simulink model "quad_control_elev8_sAttit_training"  (Simulink 8.7)
settings: Solver=FixedStepAuto  StartTime=0.0  StopTime=20  FixedStep=0.01  RelTol=1e-3
InitFcn:
  | % --- Inner loop gains --------
  | %Kp_pitch = 2.5;   Kp_roll = 2.5;    Kp_yaw = 0.4;
  | %Ki_pitch = 0.06;  Ki_roll = 0.055; Ki_yaw = 0.095;
  | %Kd_pitch = 1.25; Kd_roll = 1.25;  Kd_yaw = 1.2;
  | % --------------------------
  | 
  | % --- Outer loop gains --------
  | P_X=9.44;   I_X=0.23; D_X=2.36;
  | P_Y=9.33;   I_Y=0.18; D_Y=1.54;
  | %P_Z = 32; I_Z = 5;  D_Z = 10;
  | % --------------------------
  | 
  | % --- Saturation limits --------
  | attit_upper_limit = 10;
  | attit_lower_limit = -10;
  | 
  | pos_upper_limit = 1;
  | pos_lower_limit = -1;
  | 
  | mvel_upper_limit = 30;
  | mvel_lower_limit = 5;
  | % --------------------------
  | 
  | %gera o valor do angulo
  | %aleatoreamente para o treinamendo
  | %de posicao
  | %rand_ang = pi + (-pi-pi).*rand(1,1);
  | %rand_altur = 1 + (3-1).*rand(1,1);
  | 
  | global clientID;
  | clientID=-1;
values from neighbouring files (symbols this model uses):
  D_Z = 35.7414524229    [workspace.mat]    (also in workspace_inner.mat = 20.4994; workspace_outer.mat = 19.0535228097)
  enable_gripper = 0    [CARLA_INNER_CONTROLLERS.m]    (also in CARLA_OUTER_CONTROLLERS.m; workspace_inner.mat; workspace_outer.mat)
  I_Z = 14.6020346537    [workspace.mat]    (also in workspace_inner.mat = 22.8237; workspace_outer.mat = 43.091018381)
  P_Z = 59.4468680841    [workspace.mat]    (also in workspace_inner.mat = 26.3889; workspace_outer.mat = 57.1774186981)
  rand_ang = pi + (-pi-pi).*rand    [CARLA_OUTER_CONTROLLERS.m]    (also in workspace.mat = 2.59590225137; workspace_outer.mat = -1.93159407417)
undefined symbols (not defined in the file or in its folder): Angular, Linear, sigbuilder_block
libraries: simulink_extras x4, dspsigops x4, robotlib x3, aerolibtransform2 x1
settings Model: Creator=kleber  LastModifiedBy=kleber
settings DataIOCC: LimitDataPoints=off
settings DebuggingCC: UnderspecifiedInitializationDetection=Simplified  MergeDetectMultiDrivingBlocksExec=error  SolverPrmCheckMsg=warning
settings ConfigComp: CovSFcnEnable=off

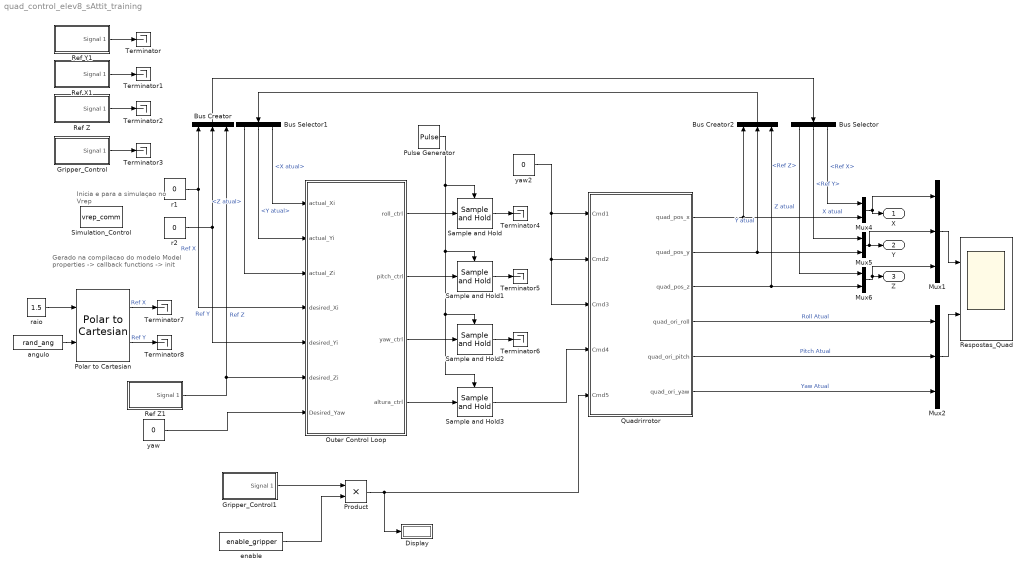
== system quad_control_elev8_sAttit_training ==
  note: Inicia e para a simulaçao no Vrep
  note: Gerado na compilacao do modelo
      | Model properties -> callback functions
      | -> init
  Bus Creator : BusCreator  Inputs=3
  Bus Creator2 : BusCreator  Inputs=3
  Bus Selector : BusSelector  OutputSignals=Ref Z,Ref Y,Ref X
  Bus Selector1 : BusSelector  OutputSignals=Z atual,Y atual,X atual
  Display : Display
  Gripper_Control : Subsystem  Tag=STV Subsys  LoadFcn=sigbuilder_block('load');  StartFcn=sigbuilder_block('start');  StopFcn=sigbuilder_block('stop');  ClipboardFcn=sigbuilder_block('clipboard');  mask(Sigbuilder block){}
      mask help: Sigbuilder GUI
      mask init:
      | if ~strcmp(get_param(bdroot(gcbh),'SimulationStatus'),'stopped') tuvar = sigbuilder_block('maskInit'); end
      settings: CopyFcn=sigbuilder_block('copy');  DeleteFcn=sigbuilder_block('delete');  ModelCloseFcn=sigbuilder_block('modelClose');  PreSaveFcn=sigbuilder_block('preSave');  PauseFcn=sigbuilder_block('pause')  ContinueFcn=sigbuilder_block('continue')  NameChangeFcn=sigbuilder_block('namechange');  OpenFcn=sigbuilder_block('open',[47.25 204 963.75 268.5 ]);  CloseFcn=sigbuilder_block('close');
      mask Display: plot(0,0,100,100,[10,10,40,40,10],[80,20,20,80,80],[40,10],[50,50], [40,27,10],[65,72,56],[40,25,25,10],[28,28,43,43]);
  Gripper_Control1 : Subsystem  Tag=STV Subsys  LoadFcn=sigbuilder_block('load');  StartFcn=sigbuilder_block('start');  StopFcn=sigbuilder_block('stop');  ClipboardFcn=sigbuilder_block('clipboard');  mask(Sigbuilder block){}
      mask help: Sigbuilder GUI
      mask init:
      | if ~strcmp(get_param(bdroot(gcbh),'SimulationStatus'),'stopped') tuvar = sigbuilder_block('maskInit'); end
      settings: CopyFcn=sigbuilder_block('copy');  DeleteFcn=sigbuilder_block('delete');  ModelCloseFcn=sigbuilder_block('modelClose');  PreSaveFcn=sigbuilder_block('preSave');  PauseFcn=sigbuilder_block('pause')  ContinueFcn=sigbuilder_block('continue')  NameChangeFcn=sigbuilder_block('namechange');  OpenFcn=sigbuilder_block('open',[47.25 138 956.25 246 ]);  CloseFcn=sigbuilder_block('close');
      mask Display: plot(0,0,100,100,[10,10,40,40,10],[80,20,20,80,80],[40,10],[50,50], [40,27,10],[65,72,56],[40,25,25,10],[28,28,43,43]);
  Mux1 : Mux  Inputs=3
  Mux2 : Mux  Inputs=3
  Mux4 : Mux  Inputs=2
  Mux5 : Mux  Inputs=2
  Mux6 : Mux  Inputs=2
  Outer Control Loop : Subsystem
  Polar to Cartesian : simulink_extras/Transformations/Polar to Cartesian
  Product : Product
  Pulse Generator : DiscretePulseGenerator  PulseType=Time based  Period=0.1  PulseWidth=10
  Quadrirrotor : Subsystem
  Ref X1 : Subsystem  Tag=STV Subsys  LoadFcn=sigbuilder_block('load');  StartFcn=sigbuilder_block('start');  StopFcn=sigbuilder_block('stop');  ClipboardFcn=sigbuilder_block('clipboard');  mask(Sigbuilder block){}
      mask help: Sigbuilder GUI
      mask init:
      | if ~strcmp(get_param(bdroot(gcbh),'SimulationStatus'),'stopped') tuvar = sigbuilder_block('maskInit'); end
      settings: CopyFcn=sigbuilder_block('copy');  DeleteFcn=sigbuilder_block('delete');  ModelCloseFcn=sigbuilder_block('modelClose');  PreSaveFcn=sigbuilder_block('preSave');  PauseFcn=sigbuilder_block('pause')  ContinueFcn=sigbuilder_block('continue')  NameChangeFcn=sigbuilder_block('namechange');  OpenFcn=sigbuilder_block('open',[62.25 205.5 902.25 227.25 ]);  CloseFcn=sigbuilder_block('close');
      mask Display: plot(0,0,100,100,[10,10,40,40,10],[80,20,20,80,80],[40,10],[50,50], [40,27,10],[65,72,56],[40,25,25,10],[28,28,43,43]);
  Ref Y1 : Subsystem  Tag=STV Subsys  LoadFcn=sigbuilder_block('load');  StartFcn=sigbuilder_block('start');  StopFcn=sigbuilder_block('stop');  ClipboardFcn=sigbuilder_block('clipboard');  mask(Sigbuilder block){}
      mask help: Sigbuilder GUI
      mask init:
      | if ~strcmp(get_param(bdroot(gcbh),'SimulationStatus'),'stopped') tuvar = sigbuilder_block('maskInit'); end
      settings: CopyFcn=sigbuilder_block('copy');  DeleteFcn=sigbuilder_block('delete');  ModelCloseFcn=sigbuilder_block('modelClose');  PreSaveFcn=sigbuilder_block('preSave');  PauseFcn=sigbuilder_block('pause')  ContinueFcn=sigbuilder_block('continue')  NameChangeFcn=sigbuilder_block('namechange');  OpenFcn=sigbuilder_block('open',[57.75 194.25 908.25 252 ]);  CloseFcn=sigbuilder_block('close');
      mask Display: plot(0,0,100,100,[10,10,40,40,10],[80,20,20,80,80],[40,10],[50,50], [40,27,10],[65,72,56],[40,25,25,10],[28,28,43,43]);
  Ref Z : Subsystem  Tag=STV Subsys  LoadFcn=sigbuilder_block('load');  StartFcn=sigbuilder_block('start');  StopFcn=sigbuilder_block('stop');  ClipboardFcn=sigbuilder_block('clipboard');  mask(Sigbuilder block){}
      mask help: Sigbuilder GUI
      mask init:
      | if ~strcmp(get_param(bdroot(gcbh),'SimulationStatus'),'stopped') tuvar = sigbuilder_block('maskInit'); end
      settings: CopyFcn=sigbuilder_block('copy');  DeleteFcn=sigbuilder_block('delete');  ModelCloseFcn=sigbuilder_block('modelClose');  PreSaveFcn=sigbuilder_block('preSave');  PauseFcn=sigbuilder_block('pause')  ContinueFcn=sigbuilder_block('continue')  NameChangeFcn=sigbuilder_block('namechange');  OpenFcn=sigbuilder_block('open',[41.25 0 973.5 255 ]);  CloseFcn=sigbuilder_block('close');
      mask Display: plot(0,0,100,100,[10,10,40,40,10],[80,20,20,80,80],[40,10],[50,50], [40,27,10],[65,72,56],[40,25,25,10],[28,28,43,43]);
  Ref Z1 : Subsystem  Tag=STV Subsys  LoadFcn=sigbuilder_block('load');  StartFcn=sigbuilder_block('start');  StopFcn=sigbuilder_block('stop');  ClipboardFcn=sigbuilder_block('clipboard');  mask(Sigbuilder block){}
      mask help: Sigbuilder GUI
      mask init:
      | if ~strcmp(get_param(bdroot(gcbh),'SimulationStatus'),'stopped') tuvar = sigbuilder_block('maskInit'); end
      settings: CopyFcn=sigbuilder_block('copy');  DeleteFcn=sigbuilder_block('delete');  ModelCloseFcn=sigbuilder_block('modelClose');  PreSaveFcn=sigbuilder_block('preSave');  PauseFcn=sigbuilder_block('pause')  ContinueFcn=sigbuilder_block('continue')  NameChangeFcn=sigbuilder_block('namechange');  OpenFcn=sigbuilder_block('open',[45 0 979.5 343.5 ]);  CloseFcn=sigbuilder_block('close');
      mask Display: plot(0,0,100,100,[10,10,40,40,10],[80,20,20,80,80],[40,10],[50,50], [40,27,10],[65,72,56],[40,25,25,10],[28,28,43,43]);
  Respostas_Quad : Scope  NumInputPorts=2
  Sample and Hold{,1..3} (4 alike) : dspsigops/Sample and Hold  trig=Rising edge  initCond=0  latchinput=off
  Simulation_Control : S-Function  FunctionName=vrep_comm  SFunctionDeploymentMode=off  EnableBusSupport=off
  Terminator{,1..8} (9 alike) : Terminator
  angulo : Constant  Value=rand_ang
  enable : Constant  Value=enable_gripper
  r1 : Constant  Value=0
  r2 : Constant  Value=0
  raio : Constant  Value=1.5
  yaw : Constant  Value=0
  yaw2 : Constant  Value=0
  X : Outport
  Y : Outport  Port=2
  Z : Outport  Port=3
  wires:
  Mux1/1 -> Respostas_Quad/1
  Mux2/1 -> Respostas_Quad/2
  Quadrirrotor/5(quad_ori_pitch) -> Mux2/2  "Pitch Atual"
  Quadrirrotor/4(quad_ori_roll) -> Mux2/1  "Roll Atual"
  Quadrirrotor/1(quad_pos_x) -> Bus Creator2/1, Mux4/2  "X atual"
  Quadrirrotor/3(quad_pos_z) -> Bus Creator2/3, Mux6/2  "Z atual"
  Quadrirrotor/6(quad_ori_yaw) -> Mux2/3  "Yaw Atual"
  yaw2/1 -> Quadrirrotor/1(Cmd1), Quadrirrotor/2(Cmd2), Quadrirrotor/3(Cmd3)
  yaw/1 -> Outer Control Loop/7(Desired_Yaw)
  Pulse Generator/1 -> Sample and Hold/Trigger, Sample and Hold2/Trigger, Sample and Hold3/Trigger, Sample and Hold1/Trigger
  Outer Control Loop/4(altura_ctrl) -> Sample and Hold3/1
  Mux4/1 -> X/1, Mux1/1
  Mux5/1 -> Y/1, Mux1/2
  Mux6/1 -> Mux1/3, Z/1
  Outer Control Loop/3(yaw_ctrl) -> Sample and Hold2/1
  Outer Control Loop/2(pitch_ctrl) -> Sample and Hold1/1
  Outer Control Loop/1(roll_ctrl) -> Sample and Hold/1
  r2/1 -> Outer Control Loop/5(desired_Yi), Bus Creator/2  "Ref Y"
  r1/1 -> Outer Control Loop/4(desired_Xi), Bus Creator/1  "Ref X"
  Quadrirrotor/2(quad_pos_y) -> Bus Creator2/2, Mux5/2  "Y atual"
  Sample and Hold3/1 -> Quadrirrotor/4(Cmd4)
  angulo/1 -> Polar to Cartesian/2
  raio/1 -> Polar to Cartesian/1
  Gripper_Control1/1(Signal 1) -> Product/1
  enable/1 -> Product/2
  Ref Y1/1(Signal 1) -> Terminator/1
  Ref X1/1(Signal 1) -> Terminator1/1
  Ref Z/1(Signal 1) -> Terminator2/1
  Gripper_Control/1(Signal 1) -> Terminator3/1
  Ref Z1/1(Signal 1) -> Outer Control Loop/6(desired_Zi), Bus Creator/3  "Ref Z"
  Bus Creator/1 -> Bus Selector/1
  Bus Selector/3 -> Mux4/1  "<Ref X>"
  Bus Selector/2 -> Mux5/1  "<Ref Y>"
  Bus Selector/1 -> Mux6/1  "<Ref Z>"
  Bus Selector1/3 -> Outer Control Loop/1(actual_Xi)  "<X atual>"
  Bus Selector1/2 -> Outer Control Loop/2(actual_Yi)  "<Y atual>"
  Bus Selector1/1 -> Outer Control Loop/3(actual_Zi)  "<Z atual>"
  Bus Creator2/1 -> Bus Selector1/1
  Product/1 -> Display/1, Quadrirrotor/5(Cmd5)
  Sample and Hold/1 -> Terminator4/1
  Sample and Hold1/1 -> Terminator5/1
  Sample and Hold2/1 -> Terminator6/1
  Polar to Cartesian/1 -> Terminator7/1  "Ref X"
  Polar to Cartesian/2 -> Terminator8/1  "Ref Y"

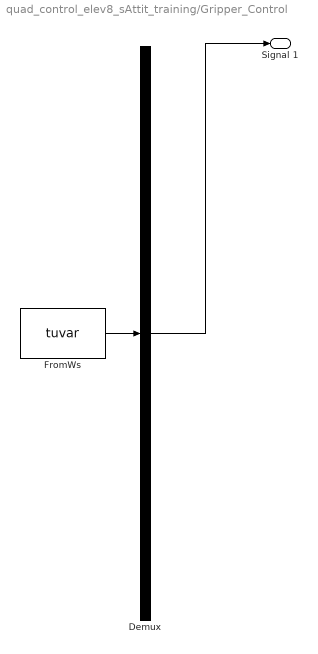
== system quad_control_elev8_sAttit_training/Gripper_Control ==
  Demux : Demux  Tag=STV Demux  Outputs=1
  FromWs : FromWorkspace  Tag=STV FromWs  VariableName=tuvar  SampleTime=0  SigBuilderData=DataTag0  VnvData=DataTag1
      SigBuilderData=|
      | common.afterFinalStr = 'Extrapolate'
      | common.sampleTime = 0
      | dataSet.timeRange = [0 250]
      | dataSet.name = 'Group 1'
      | sbobj.Name = 'Signal Builder'
      | sbobj.Groups.Name = 'Group 1'
      | sbobj.Groups.Signals.Name = 'Signal 1'
      | sbobj.Groups.Signals.XData = [0 35 35 100 100 155 155 220 220 250]
      | sbobj.Groups.Signals.YData = [0 0 1 1 0 0 1 1 0 0]
      | sbobj.Groups.TimeRange = [0 250]
  Signal 1 : Outport  Tag=STV Outport
  wires:
  FromWs/1 -> Demux/1
  Demux/1 -> Signal 1/1

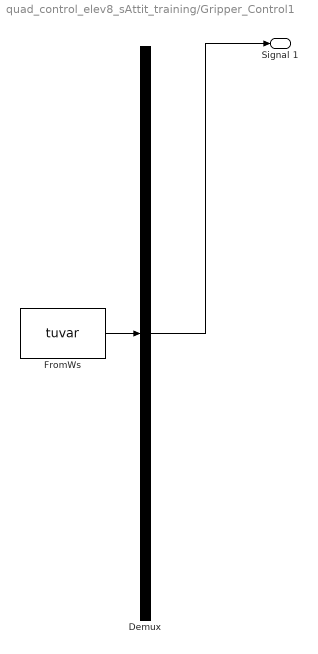
== system quad_control_elev8_sAttit_training/Gripper_Control1 ==
  Demux : Demux  Tag=STV Demux  Outputs=1
  FromWs : FromWorkspace  Tag=STV FromWs  VariableName=tuvar  SampleTime=0  SigBuilderData=DataTag2  VnvData=DataTag3
      SigBuilderData=|
      | common.afterFinalStr = 'Extrapolate'
      | common.sampleTime = 0
      | dataSet.timeRange = [0 40]
      | dataSet.name = 'Group 1'
      | sbobj.Name = 'Signal Builder'
      | sbobj.Groups.Name = 'Group 1'
      | sbobj.Groups.Signals.Name = 'Signal 1'
      | sbobj.Groups.Signals.XData = [0 22.5 22.5 40]
      | sbobj.Groups.Signals.YData = [1 1 0 0]
      | sbobj.Groups.TimeRange = [0 40]
  Signal 1 : Outport  Tag=STV Outport
  wires:
  Demux/1 -> Signal 1/1
  FromWs/1 -> Demux/1

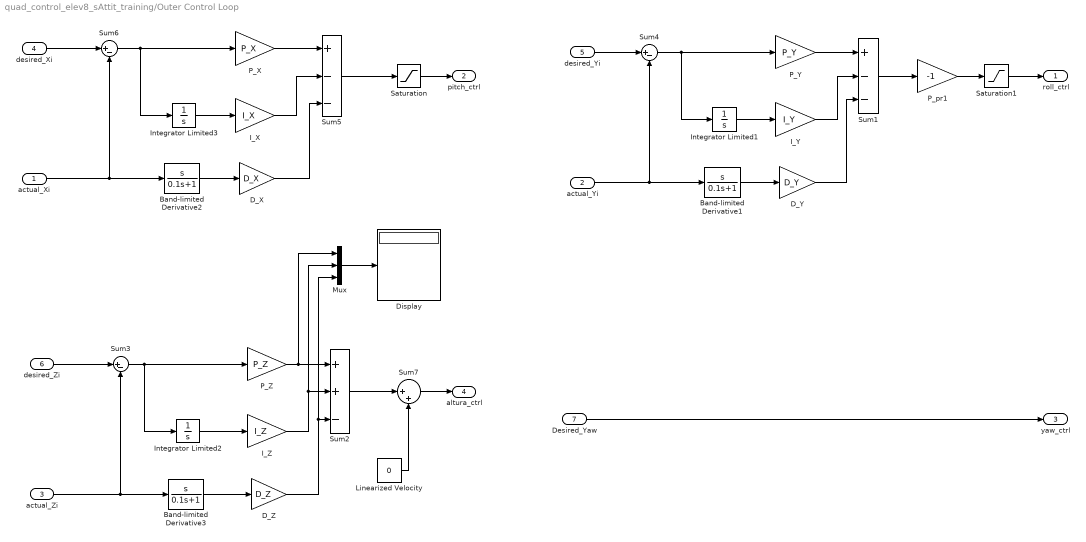
== system quad_control_elev8_sAttit_training/Outer Control Loop ==
  actual_Xi : Inport
  actual_Yi : Inport  Port=2
  actual_Zi : Inport  Port=3
  desired_Xi : Inport  Port=4
  desired_Yi : Inport  Port=5
  desired_Zi : Inport  Port=6
  Desired_Yaw : Inport  Port=7
  Band-limited Derivative1 : TransferFcn  Numerator=[1 0]  Denominator=[0.1 1]
  Band-limited Derivative2 : TransferFcn  Numerator=[1 0]  Denominator=[0.1 1]
  Band-limited Derivative3 : TransferFcn  Numerator=[1 0]  Denominator=[0.1 1]
  D_X : Gain  Gain=D_X
  D_Y : Gain  Gain=D_Y
  D_Z : Gain  Gain=D_Z
  Display : Display
  I_X : Gain  Gain=I_X
  I_Y : Gain  Gain=I_Y
  I_Z : Gain  Gain=I_Z
  Integrator Limited1 : Integrator  LimitOutput=on  UpperSaturationLimit=0.5  LowerSaturationLimit=-0.5
  Integrator Limited2 : Integrator  LimitOutput=on  UpperSaturationLimit=10  LowerSaturationLimit=0
  Integrator Limited3 : Integrator  LimitOutput=on  UpperSaturationLimit=0.5  LowerSaturationLimit=-0.5
  Linearized Velocity : Constant  Value=0
  Mux : Mux  Inputs=3
  P_X : Gain  Gain=P_X
  P_Y : Gain  Gain=P_Y
  P_Z : Gain  Gain=P_Z
  P_pr1 : Gain  Gain=-1
  Saturation : Saturate  UpperLimit=2  LowerLimit=-2
  Saturation1 : Saturate  UpperLimit=2  LowerLimit=-2
  Sum1 : Sum  Inputs=+--
  Sum2 : Sum  Inputs=++-
  Sum3 : Sum  Inputs=|+-
  Sum4 : Sum  Inputs=|+-
  Sum5 : Sum  Inputs=+--
  Sum6 : Sum  Inputs=|+-
  Sum7 : Sum  Inputs=|++
  roll_ctrl : Outport
  pitch_ctrl : Outport  Port=2
  yaw_ctrl : Outport  Port=3
  altura_ctrl : Outport  Port=4
  wires:
  Sum7/1 -> altura_ctrl/1
  Desired_Yaw/1 -> yaw_ctrl/1
  Sum1/1 -> P_pr1/1
  Sum2/1 -> Sum7/1
  Linearized Velocity/1 -> Sum7/2
  Sum5/1 -> Saturation/1
  Saturation/1 -> pitch_ctrl/1
  P_pr1/1 -> Saturation1/1
  Saturation1/1 -> roll_ctrl/1
  Mux/1 -> Display/1
  Sum3/1 -> Integrator Limited2/1, P_Z/1
  P_Z/1 -> Mux/1, Sum2/1
  D_Z/1 -> Mux/3, Sum2/3
  Band-limited Derivative3/1 -> D_Z/1
  I_Z/1 -> Mux/2, Sum2/2
  Sum6/1 -> Integrator Limited3/1, P_X/1
  Integrator Limited3/1 -> I_X/1
  P_X/1 -> Sum5/1
  D_X/1 -> Sum5/3
  actual_Xi/1 -> Band-limited Derivative2/1, Sum6/2
  Band-limited Derivative2/1 -> D_X/1
  desired_Xi/1 -> Sum6/1
  I_X/1 -> Sum5/2
  Integrator Limited2/1 -> I_Z/1
  Sum4/1 -> Integrator Limited1/1, P_Y/1
  Integrator Limited1/1 -> I_Y/1
  P_Y/1 -> Sum1/1
  D_Y/1 -> Sum1/3
  actual_Yi/1 -> Sum4/2, Band-limited Derivative1/1
  Band-limited Derivative1/1 -> D_Y/1
  desired_Yi/1 -> Sum4/1
  I_Y/1 -> Sum1/2
  actual_Zi/1 -> Sum3/2, Band-limited Derivative3/1
  desired_Zi/1 -> Sum3/1

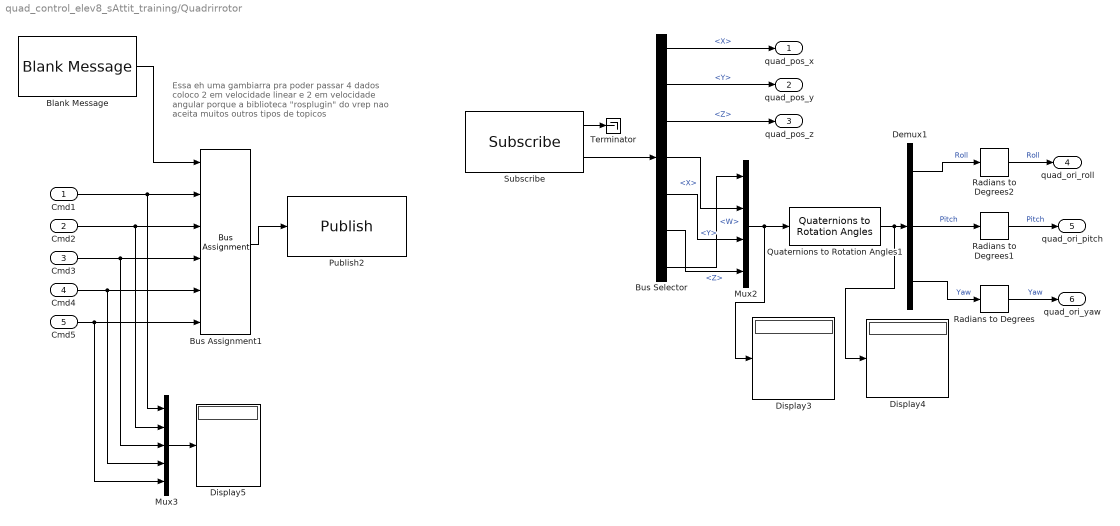
== system quad_control_elev8_sAttit_training/Quadrirrotor ==
  note: Essa eh uma gambiarra pra poder passar 4 dados coloco 2 em velocidade linear e 2 em velocidade angular porque a biblioteca "rosplugin" do vrep nao aceita muitos outros tipos de topicos
  Cmd1 : Inport
  Cmd2 : Inport  Port=2
  Cmd3 : Inport  Port=3
  Cmd4 : Inport  Port=4
  Cmd5 : Inport  Port=5
  Blank Message : robotlib/Blank Message  SourceLibraryInfo=This block requires Robotics System Toolbox  messageType=geometry_msgs/Twist  SampleTime=inf
  Bus Assignment1 : BusAssignment  DialogController=Simulink.DDGSource_BusAssignment  AssignedSignals=Linear.X,Linear.Y,Angular.X,Angular.Y,Angular.Z
  Bus Selector : BusSelector  OutputSignals=Pose.Position.X,Pose.Position.Y,Pose.Position.Z,Pose.Orientation.X,Pose.Orientation.Y,Pose.Orientation.Z,Pose.Orientation.W
  Demux1 : Demux  Outputs=3
  Display3 : Display
  Display4 : Display
  Display5 : Display
  Mux2 : Mux
  Mux3 : Mux  Inputs=5
  Publish2 : robotlib/Publish  SourceLibraryInfo=This block requires Robotics System Toolbox  topicSource=Select from ROS network  topic=/control_signals  messageType=geometry_msgs/Twist  messageQueueLength=105
  Quaternions to Rotation Angles1 : aerolibtransform2/Quaternions to Rotation Angles  rotationOrder=XYZ
  Radians to Degrees : simulink_extras/Transformations/Radians to Degrees
  Radians to Degrees1 : simulink_extras/Transformations/Radians to Degrees
  Radians to Degrees2 : simulink_extras/Transformations/Radians to Degrees
  Subscribe : robotlib/Subscribe  SourceLibraryInfo=This block requires Robotics System Toolbox  topicSource=Select from ROS network  topic=/quad_pos_ang  messageType=geometry_msgs/PoseStamped  sampleTime=-1  messageQueueLength=51
  Terminator : Terminator
  quad_pos_x : Outport
  quad_pos_y : Outport  Port=2
  quad_pos_z : Outport  Port=3
  quad_ori_roll : Outport  Port=4
  quad_ori_pitch : Outport  Port=5
  quad_ori_yaw : Outport  Port=6
  wires:
  Cmd1/1 -> Mux3/1, Bus Assignment1/2
  Bus Selector/1 -> quad_pos_x/1  "<X>"
  Bus Selector/2 -> quad_pos_y/1  "<Y>"
  Bus Selector/3 -> quad_pos_z/1  "<Z>"
  Radians to Degrees2/1 -> quad_ori_roll/1  "Roll"
  Radians to Degrees1/1 -> quad_ori_pitch/1  "Pitch"
  Radians to Degrees/1 -> quad_ori_yaw/1  "Yaw"
  Demux1/3 -> Radians to Degrees/1  "Yaw"
  Demux1/2 -> Radians to Degrees1/1  "Pitch"
  Demux1/1 -> Radians to Degrees2/1  "Roll"
  Bus Assignment1/1 -> Publish2/1
  Blank Message/1 -> Bus Assignment1/1
  Subscribe/2 -> Bus Selector/1
  Subscribe/1 -> Terminator/1
  Bus Selector/5 -> Mux2/3  "<Y>"
  Bus Selector/6 -> Mux2/4  "<Z>"
  Bus Selector/7 -> Mux2/1  "<W>"
  Mux2/1 -> Quaternions to Rotation Angles1/1, Display3/1
  Bus Selector/4 -> Mux2/2  "<X>"
  Cmd3/1 -> Mux3/3, Bus Assignment1/4
  Cmd4/1 -> Bus Assignment1/5, Mux3/4
  Quaternions to Rotation Angles1/1 -> Display4/1, Demux1/1
  Mux3/1 -> Display5/1
  Cmd2/1 -> Mux3/2, Bus Assignment1/3
  Cmd5/1 -> Bus Assignment1/6, Mux3/5

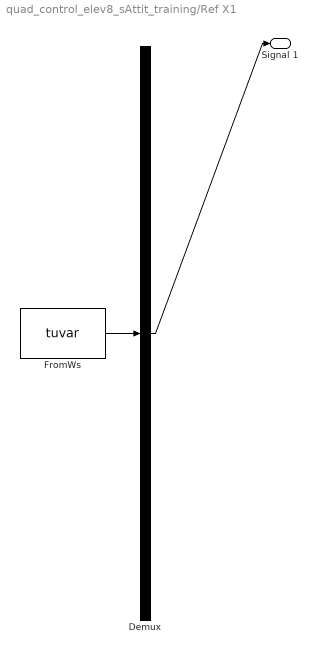
== system quad_control_elev8_sAttit_training/Ref X1 ==
  Demux : Demux  Tag=STV Demux  Outputs=1
  FromWs : FromWorkspace  Tag=STV FromWs  VariableName=tuvar  SampleTime=0  SigBuilderData=DataTag4  VnvData=DataTag5
      SigBuilderData=|
      | common.afterFinalStr = 'Extrapolate'
      | common.sampleTime = 0
      | dataSet.timeRange = [0 250]
      | dataSet.name = 'Group 1'
      | sbobj.Name = 'Signal Builder'
      | sbobj.Groups.Name = 'Group 1'
      | sbobj.Groups.Signals.Name = 'Signal 1'
      | sbobj.Groups.Signals.XData = [0 10 110 130 250]
      | sbobj.Groups.Signals.YData = [0 1 1 1.5 1.5]
      | sbobj.Groups.TimeRange = [0 250]
  Signal 1 : Outport  Tag=STV Outport
  wires:
  FromWs/1 -> Demux/1
  Demux/1 -> Signal 1/1

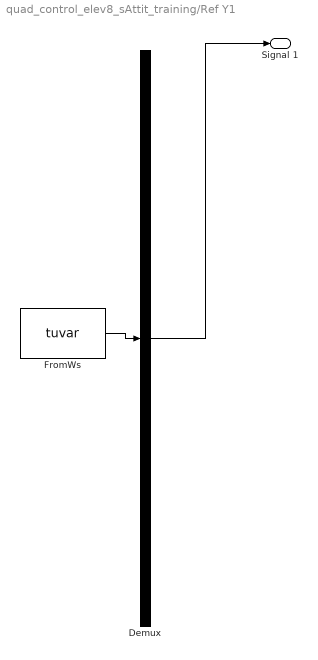
== system quad_control_elev8_sAttit_training/Ref Y1 ==
  Demux : Demux  Tag=STV Demux  Outputs=1
  FromWs : FromWorkspace  Tag=STV FromWs  VariableName=tuvar  SampleTime=0  SigBuilderData=DataTag6  VnvData=DataTag7
      SigBuilderData=|
      | common.afterFinalStr = 'Extrapolate'
      | common.sampleTime = 0
      | dataSet.timeRange = [0 250]
      | dataSet.name = 'Group 1'
      | sbobj.Name = 'Signal Builder'
      | sbobj.Groups.Name = 'Group 1'
      | sbobj.Groups.Signals.Name = 'Signal 1'
      | sbobj.Groups.Signals.XData = [0 10 50 70 105 130 170 190 250]
      | sbobj.Groups.Signals.YData = [0 0.5 0.5 2.5 2.5 0.5 0.5 2.5 2.5]
      | sbobj.Groups.TimeRange = [0 250]
  Signal 1 : Outport  Tag=STV Outport
  wires:
  Demux/1 -> Signal 1/1
  FromWs/1 -> Demux/1

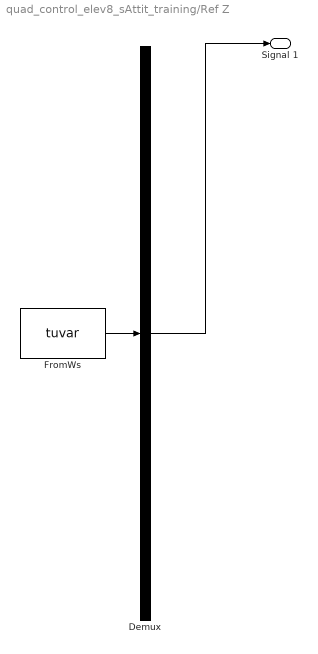
== system quad_control_elev8_sAttit_training/Ref Z ==
  Demux : Demux  Tag=STV Demux  Outputs=1
  FromWs : FromWorkspace  Tag=STV FromWs  VariableName=tuvar  SampleTime=0  SigBuilderData=DataTag8  VnvData=DataTag9
      SigBuilderData=|
      | common.afterFinalStr = 'Extrapolate'
      | common.sampleTime = 0
      | dataSet.timeRange = [0 250]
      | dataSet.name = 'Group 1'
      | sbobj.Name = 'Signal Builder'
      | sbobj.Groups.Name = 'Group 1'
      | sbobj.Groups.Signals.Name = 'Signal 1'
      | sbobj.Groups.Signals.XData = [0 1 20 35 40 55 80 95 100 115 140 155 160 175 200 215 220 235 250]
      | sbobj.Groups.Signals.YData = [0 0.5 0.5 0.14 0.14 0.5 0.5 0.15 0.15 0.5 0.5 0.15 0.15 0.5 0.5 0.15 0.15 0.5 0.5]
      | sbobj.Groups.TimeRange = [0 250]
  Signal 1 : Outport  Tag=STV Outport
  wires:
  Demux/1 -> Signal 1/1
  FromWs/1 -> Demux/1

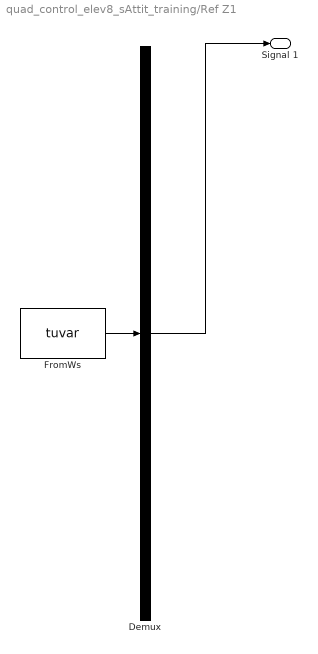
== system quad_control_elev8_sAttit_training/Ref Z1 ==
  Demux : Demux  Tag=STV Demux  Outputs=1
  FromWs : FromWorkspace  Tag=STV FromWs  VariableName=tuvar  SampleTime=0  SigBuilderData=DataTag10  VnvData=DataTag11
      SigBuilderData=|
      | common.afterFinalStr = 'Extrapolate'
      | common.sampleTime = 0
      | dataSet.timeRange = [0 40]
      | dataSet.name = 'Group 1'
      | sbobj.Name = 'Signal Builder'
      | sbobj.Groups.Name = 'Group 1'
      | sbobj.Groups.Signals.Name = 'Signal 1'
      | sbobj.Groups.Signals.XData = [0 10 20 22.5 25 30 40]
      | sbobj.Groups.Signals.YData = [0.12 1 1 0.15 0.15 0.5 0.5]
      | sbobj.Groups.TimeRange = [0 40]
  Signal 1 : Outport  Tag=STV Outport
  wires:
  FromWs/1 -> Demux/1
  Demux/1 -> Signal 1/1
